simulink model "active_vibration_damping_lab_model"  (R2016a)
settings: Solver=FixedStepAuto  StartTime=0.0  StopTime=inf  RelTol=1e-3
libraries: legoev3lib x2
settings Model: SimulationMode=external  ExtModeTrigDuration=2  Creator=Zehra Fatih  LastModifiedBy=Zehra Fatih
settings SolverCC: PositivePriorityOrder=on  AutoInsertRateTranBlk=on
settings OptimizationCC: OptimizeModelRefInitCode=on  LifeSpan=1  MaxStackSize=64
settings HardwareCC: ProdBitPerPointer=32  ProdLargestAtomicInteger=Long  ProdWordSize=32  ProdHWDeviceType=ARM Compatible->ARM 9
settings RTWCC: SystemTargetFile=ert.tlc  HardwareBoard=LEGO MINDSTORMS EV3  TemplateMakefile=ert_default_tmf  GenerateReport=on  Toolchain=Sourcery G++ Lite v2009q3  IncludeHyperlinkInReport=on  LaunchReport=on  GenerateTraceInfo=on  GenerateTraceReport=on  GenerateTraceReportSl=on  GenerateTraceReportSf=on  GenerateTraceReportEml=on
settings CodeAppCC: ForceParamTrailComments=on  IgnoreCustomStorageClasses=off  OperatorAnnotations=on  SimulinkDataObjDesc=on  SFDataObjDesc=on  MATLABFcnDesc=on  MangleLength=10  InsertBlockDesc=on  MATLABSourceComments=on
settings ERTTargetCC: SupportContinuousTime=on  SupportVariableSizeSignals=on  ExtMode=on  ExtModeMexArgs='192.168.2.102' 0 17725

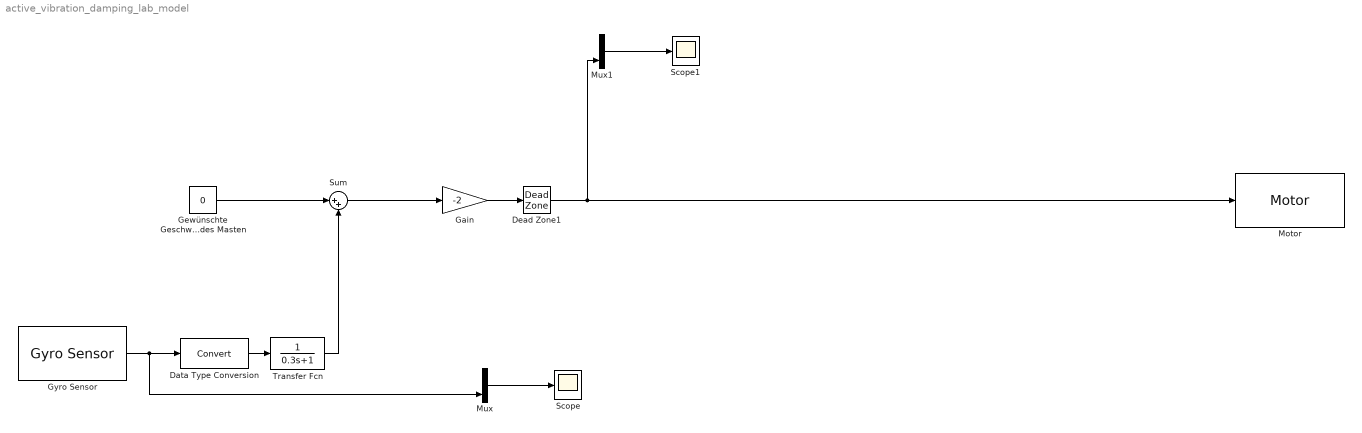
== system active_vibration_damping_lab_model ==
  Data Type Conversion : DataTypeConversion
  Dead Zone1 : DeadZone  LowerValue=-20  UpperValue=20  SaturateOnIntegerOverflow=on
  Gain : Gain  Gain=-2
  Gewünschte Geschwindigkeit des Masten : Constant  Value=0
  Gyro Sensor : legoev3lib/Gyro Sensor  portNumber=4  sampleTime=0.01
  Motor : legoev3lib/Motor  sportNumber=A  sstopAction=Brake
  Mux : Mux  Inputs=2
  Mux1 : Mux  Inputs=2
  Scope : Scope
  Scope1 : Scope
  Sum : Sum  Inputs=|++
  Transfer Fcn : TransferFcn  Denominator=[0.3 1]
  wires:
  Mux/1 -> Scope/1
  Gewünschte Geschwindigkeit des Masten/1 -> Sum/1
  Mux1/1 -> Scope1/1
  Gyro Sensor/1 -> Mux/2, Data Type Conversion/1
  Sum/1 -> Gain/1
  Gain/1 -> Dead Zone1/1
  Dead Zone1/1 -> Mux1/2, Motor/1
  Data Type Conversion/1 -> Transfer Fcn/1
  Transfer Fcn/1 -> Sum/2
